simulink model "simulacao_discreto"  (R2021b)
settings: Solver=VariableStepAuto  StartTime=0.0  StopTime=5  RelTol=1e-3
values from neighbouring files (symbols this model uses):
  sys_d = c2d(sys_ss,Ts,'zoh')    [ganhos_lqr_discreto.m]
undefined symbols (not defined in the file or in its folder): Kd
settings Model: Creator=marco  LastModifiedBy=marco

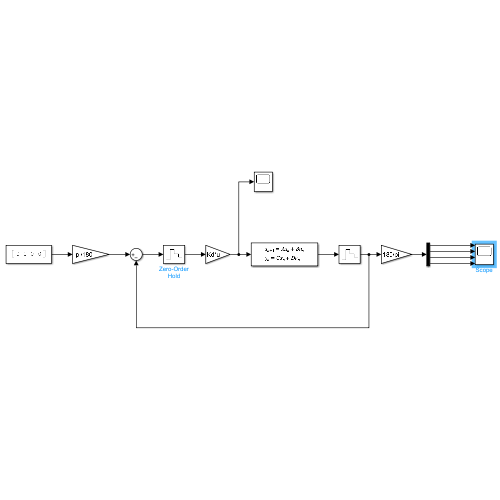
[thumbnail: Simulink's stored preview of the top-level diagram]
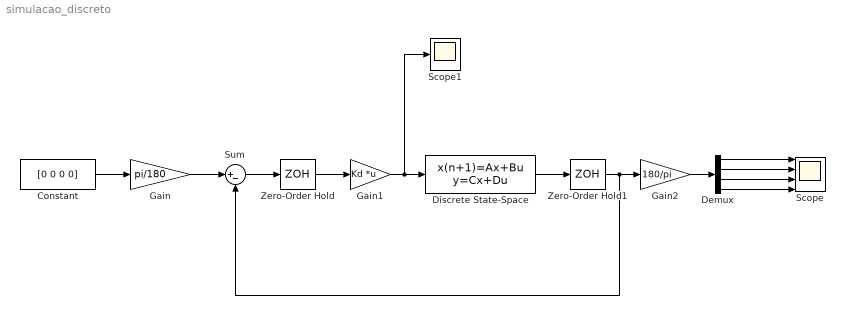
== system simulacao_discreto ==
  Constant : Constant  Value=[0 0 0 0]
  Demux : Demux
  Discrete State-Space : DiscreteStateSpace  A=sys_d.A  B=sys_d.B  C=sys_d.C  D=sys_d.D  InitialCondition=[0,5*pi/180,0,0]  SampleTime=0.06
  Gain : Gain  Gain=pi/180
  Gain1 : Gain  Gain=Kd  Multiplication=Matrix(K*u)
  Gain2 : Gain  Gain=180/pi
  Scope : Scope  NumInputPorts=4
  Scope1 : Scope
  Sum : Sum  Inputs=|+-
  Zero-Order Hold : ZeroOrderHold  SampleTime=0.06
  Zero-Order Hold1 : ZeroOrderHold  SampleTime=0.06
  wires:
  Constant/1 -> Gain/1
  Gain/1 -> Sum/1
  Sum/1 -> Zero-Order Hold/1
  Zero-Order Hold/1 -> Gain1/1
  Gain1/1 -> Discrete State-Space/1, Scope1/1
  Zero-Order Hold1/1 -> Sum/2, Gain2/1
  Demux/3 -> Scope/3
  Gain2/1 -> Demux/1
  Demux/1 -> Scope/1
  Demux/2 -> Scope/2
  Demux/4 -> Scope/4
  Discrete State-Space/1 -> Zero-Order Hold1/1
